simulink model "PIDControllerThetap"  (R2017a)
settings: Solver=VariableStepAuto  StartTime=0.0  StopTime=10.0  RelTol=1e-3
settings Model: Creator=DF_Local  LastModifiedBy=DF_Local

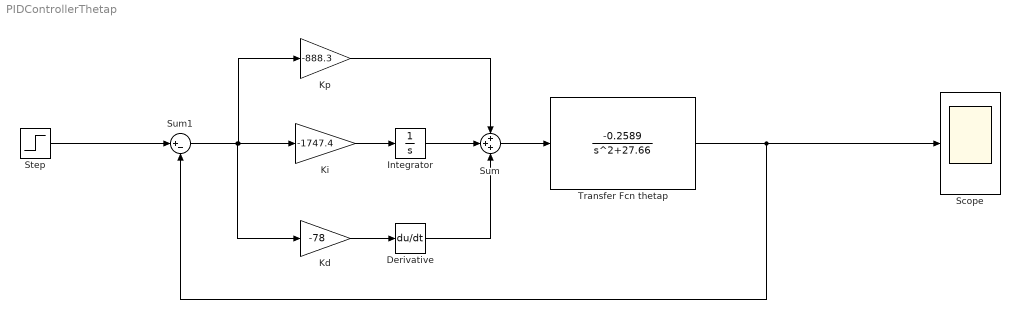
== system PIDControllerThetap ==
  Derivative : Derivative
  Integrator : Integrator
  Kd : Gain  Gain=-78
  Ki : Gain  Gain=-1747.4
  Kp : Gain  Gain=-888.3
  Scope : Scope
  Step : Step  Time=0  SampleTime=0
  Sum : Sum  Inputs=+++
  Sum1 : Sum  Inputs=|+-
  Transfer Fcn thetap : TransferFcn  Numerator=[-0.2589]  Denominator=[1 0 27.66]
  wires:
  Sum1/1 -> Ki/1, Kp/1, Kd/1
  Kd/1 -> Derivative/1
  Kp/1 -> Sum/1
  Sum/1 -> Transfer Fcn thetap/1
  Transfer Fcn thetap/1 -> Scope/1, Sum1/2
  Step/1 -> Sum1/1
  Derivative/1 -> Sum/3
  Integrator/1 -> Sum/2
  Ki/1 -> Integrator/1
